simulink model "Msimlab3parte3"  (R2021a)
settings: Solver=VariableStepAuto  StartTime=0.0  StopTime=10  MaxStep=1e-4  RelTol=1e-3
values from neighbouring files (symbols this model uses):
  b = -0.8    [p3.m]
libraries: simulink x3
settings Model: Creator=danie  LastModifiedBy=ruipe
settings SolverCC: ZeroCrossAlgorithm=Adaptive  AlgebraicLoopSolver=TrustRegion
settings DebuggingCC: IgnoredZcDiagnostic=none  SFMachineParentedDataDiag=warning

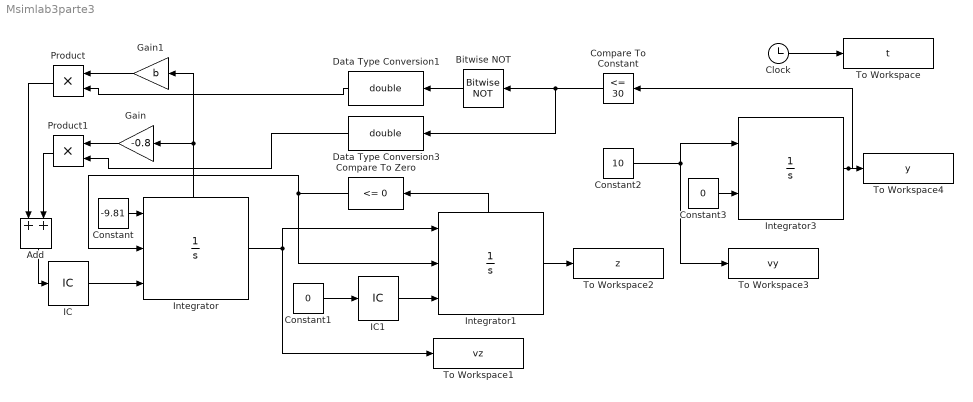
== system Msimlab3parte3 ==
  Add : Sum
  Bitwise NOT : simulink/Logic and Bit Operations/Bitwise Operator  logicop=NOT  UseBitMask=off  BitMask=bin2dec('11011001')  BitMaskRealWorld=Stored Integer
  Clock : Clock
  Compare To Constant : simulink/Logic and Bit Operations/Compare To Constant  relop=<=  const=30  OutDataTypeStr=boolean
  Compare To Zero : simulink/Logic and Bit Operations/Compare To Zero  relop=<=  OutDataTypeStr=boolean
  Constant : Constant  Description=Gravidade  Value=-9.81
      settings: AttributesFormatString=Gravidade
  Constant1 : Constant  Description=Pavimento  Value=0
      settings: AttributesFormatString=Pavimento
  Constant2 : Constant  Description=Gravidade  Value=10  OutDataTypeStr=double
      settings: AttributesFormatString=Velocidade inicial y
  Constant3 : Constant  Description=Gravidade  Value=0
  Data Type Conversion1 : DataTypeConversion  OutDataTypeStr=double
  Data Type Conversion3 : DataTypeConversion  OutDataTypeStr=double
  Gain : Gain  Description=Elasticidade da bola  Gain=-0.8
      settings: AttributesFormatString=Elasticidade da bola
  Gain1 : Gain  Description=Elasticidade da bola  Gain=b
      settings: AttributesFormatString=Elasticidade da bola
  IC : InitialCondition  Description=Velocidade inicial  Value=0
      settings: AttributesFormatString=Velocidade inicial z
  IC1 : InitialCondition  Description=Posição inicial  Value=10
      settings: AttributesFormatString=Posição inicial z
  Integrator : Integrator  ExternalReset=level hold  InitialConditionSource=external  ShowStatePort=on
      settings: AttributesFormatString=Velocidade z
  Integrator1 : Integrator  ExternalReset=rising  InitialConditionSource=external  LimitOutput=on  ShowStatePort=on
      settings: AttributesFormatString=Posição z
  Integrator3 : Integrator  InitialConditionSource=external
      settings: AttributesFormatString=Posição y
  Product : Product
  Product1 : Product
  To Workspace : ToWorkspace  VariableName=t  SaveFormat=Timeseries  SampleTime=-1
      settings: Save2DSignal=2-D array (concatenate along first dimension)
  To Workspace1 : ToWorkspace  VariableName=vz  SaveFormat=Timeseries  SampleTime=-1
      settings: Save2DSignal=2-D array (concatenate along first dimension)
  To Workspace2 : ToWorkspace  VariableName=z  SaveFormat=Timeseries  SampleTime=-1
      settings: Save2DSignal=2-D array (concatenate along first dimension)
  To Workspace3 : ToWorkspace  VariableName=vy  SaveFormat=Timeseries  SampleTime=-1
      settings: Save2DSignal=2-D array (concatenate along first dimension)
  To Workspace4 : ToWorkspace  VariableName=y  SaveFormat=Timeseries  SampleTime=-1
      settings: Save2DSignal=2-D array (concatenate along first dimension)
  wires:
  Integrator1/1 -> To Workspace2/1
  Integrator1/State -> Compare To Zero/1
  Compare To Zero/1 -> Integrator/2, Integrator1/2
  Constant1/1 -> IC1/1
  IC1/1 -> Integrator1/3
  IC/1 -> Integrator/3
  Integrator/1 -> Integrator1/1, To Workspace1/1
  Clock/1 -> To Workspace/1
  Constant2/1 -> Integrator3/1, To Workspace3/1
  Integrator3/1 -> Compare To Constant/1, To Workspace4/1
  Constant/1 -> Integrator/1
  Integrator/State -> Gain1/1, Gain/1
  Compare To Constant/1 -> Data Type Conversion3/1, Bitwise NOT/1
  Product1/1 -> Add/2
  Add/1 -> IC/1
  Constant3/1 -> Integrator3/2
  Product/1 -> Add/1
  Data Type Conversion1/1 -> Product/2
  Bitwise NOT/1 -> Data Type Conversion1/1
  Gain1/1 -> Product/1
  Data Type Conversion3/1 -> Product1/2
  Gain/1 -> Product1/1
